simulink model "conv_coder"  (R2017b)
settings: Solver=VariableStepAuto  StartTime=0.0  StopTime=999999  RelTol=1e-3
libraries: commcnvcod2 x4, commsink2 x2, commutil2 x2, commrandsrc3 x1, commchan3 x1
settings Model: Creator=adgp97  LastModifiedBy=adgp97

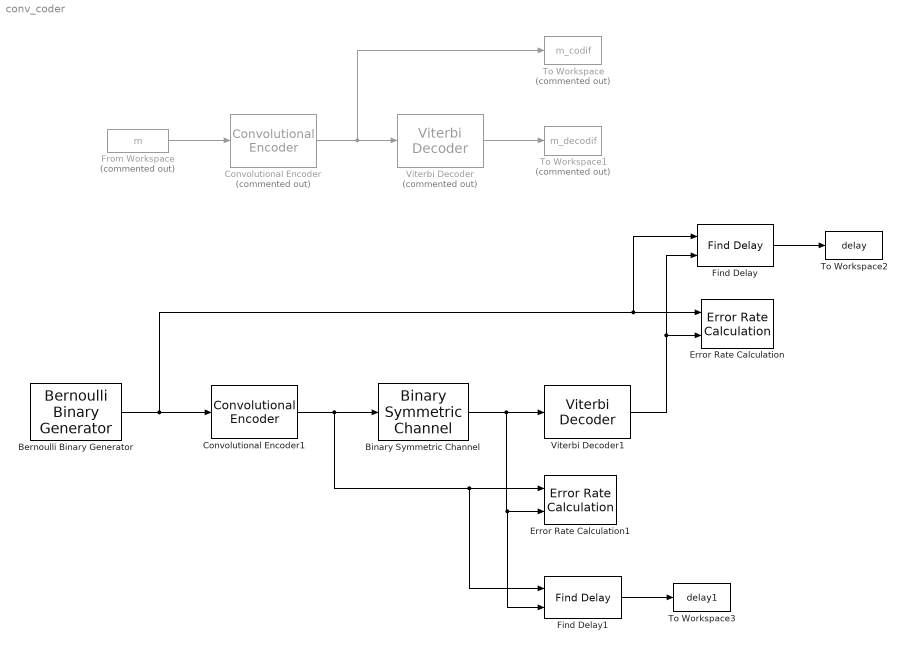
== system conv_coder ==
  Bernoulli Binary Generator : commrandsrc3/Bernoulli Binary Generator  ProbabilityOfZero=0.5  SeedSource=Auto  Seed=0  SampleTime=1  SamplesPerFrame=1  OutputDataType=double  SimulateUsing=Interpreted execution
  Binary Symmetric Channel : commchan3/Binary Symmetric Channel  P=0.1  s=71  E=off  outDtype=double
      settings: SourceProductName=Communications System Toolbox  SourceProductBaseCode=CM
  Convolutional Encoder : commcnvcod2/Convolutional Encoder  Commented=on  trellis=t  opMode=Continuous  DelayedResetAction=off  hasIniStPort=off  hasFinStPort=off  usePuncVector=off  punctureVector=[1; 1; 0; 1; 0; 1]  reset=Unused parameter value
      settings: SourceProductName=Communications System Toolbox  SourceProductBaseCode=CM
  Convolutional Encoder1 : commcnvcod2/Convolutional Encoder  trellis=t  opMode=Continuous  DelayedResetAction=off  hasIniStPort=off  hasFinStPort=off  usePuncVector=off  punctureVector=[1; 1; 0; 1; 0; 1]  reset=Unused parameter value
      settings: SourceProductName=Communications System Toolbox  SourceProductBaseCode=CM
  Error Rate Calculation : commsink2/Error Rate Calculation  N=3  st_delay=0  cp_mode=Entire frame  subframe=[]  PMode=Workspace  WsName=ErrorVec2  RsMode2=off  stop=on  numErr=1000  maxBits=1e6
  Error Rate Calculation1 : commsink2/Error Rate Calculation  N=0  st_delay=0  cp_mode=Entire frame  subframe=[]  PMode=Workspace  WsName=ErrorVec1  RsMode2=off  stop=on  numErr=1000  maxBits=1e6
  Find Delay : commutil2/Find Delay  corrLength=200  chgSigOP=off  stopUpdate=on  numConstDelay=3
      settings: SourceProductName=Communications System Toolbox  SourceProductBaseCode=CM
  Find Delay1 : commutil2/Find Delay  corrLength=200  chgSigOP=off  stopUpdate=on  numConstDelay=3
      settings: SourceProductName=Communications System Toolbox  SourceProductBaseCode=CM
  From Workspace : FromWorkspace  Commented=on  VariableName=m  SampleTime=0
  To Workspace : ToWorkspace  Commented=on  VariableName=m_codif  SampleTime=-1
      settings: Save2DSignal=2-D array (concatenate along first dimension)
  To Workspace1 : ToWorkspace  Commented=on  VariableName=m_decodif  SampleTime=-1
  To Workspace2 : ToWorkspace  VariableName=delay  SampleTime=-1
      settings: Save2DSignal=2-D array (concatenate along first dimension)
  To Workspace3 : ToWorkspace  VariableName=delay1  SampleTime=-1
      settings: Save2DSignal=2-D array (concatenate along first dimension)
  Viterbi Decoder : commcnvcod2/Viterbi Decoder  Commented=on  trellis=t  isPunctured=off  punctureVector=[1; 1; 0; 1; 0; 1]  erasures=off  dectype=Hard decision  nsdecb=4  runSigValErrCheck=on  tbdepth=3  opmode=Truncated  reset=off  delayedResetAction=off  smWordLength=16  outDataType=Inherit via internal rule
      settings: SourceProductName=Communications System Toolbox  SourceProductBaseCode=CM
  Viterbi Decoder1 : commcnvcod2/Viterbi Decoder  trellis=t  isPunctured=off  punctureVector=[1; 1; 0; 1; 0; 1]  erasures=off  dectype=Hard decision  nsdecb=4  runSigValErrCheck=on  tbdepth=3  opmode=Continuous  reset=off  delayedResetAction=off  smWordLength=16  outDataType=Inherit via internal rule
      settings: SourceProductName=Communications System Toolbox  SourceProductBaseCode=CM
  wires:
  From Workspace/1 -> Convolutional Encoder/1
  Convolutional Encoder/1 -> To Workspace/1, Viterbi Decoder/1
  Viterbi Decoder/1 -> To Workspace1/1
  Bernoulli Binary Generator/1 -> Find Delay/1, Error Rate Calculation/1, Convolutional Encoder1/1
  Binary Symmetric Channel/1 -> Find Delay1/2, Error Rate Calculation1/2, Viterbi Decoder1/1
  Convolutional Encoder1/1 -> Find Delay1/1, Error Rate Calculation1/1, Binary Symmetric Channel/1
  Viterbi Decoder1/1 -> Find Delay/2, Error Rate Calculation/2
  Find Delay/1 -> To Workspace2/1
  Find Delay1/1 -> To Workspace3/1
